simulink model "usrmpc"  (R2018b)
settings: Solver=VariableStepAuto  StartTime=0.0  StopTime=10.0  RelTol=1e-3
settings Model: Creator=dongdaming  LastModifiedBy=dongdaming

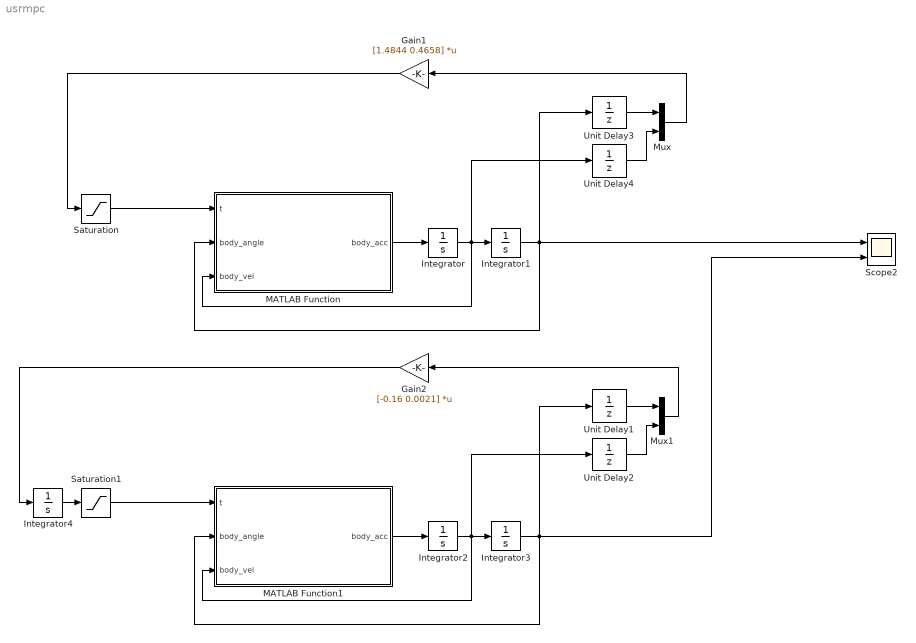
== system usrmpc ==
  Gain1 : Gain  Gain=[1.4844 0.4658]  Multiplication=Matrix(K*u)
  Gain2 : Gain  Gain=[-0.16 0.0021]  Multiplication=Matrix(K*u)
  Integrator : Integrator
  Integrator1 : Integrator  InitialCondition=pi/3  LimitOutput=on  UpperSaturationLimit=pi  LowerSaturationLimit=-pi
  Integrator2 : Integrator
  Integrator3 : Integrator  InitialCondition=pi/3  LimitOutput=on  UpperSaturationLimit=pi  LowerSaturationLimit=-pi
  Integrator4 : Integrator
  MATLAB Function : MATLAB Function  TreatAsAtomicUnit=on
  MATLAB Function1 : MATLAB Function  TreatAsAtomicUnit=on
  Mux : Mux  Inputs=2
  Mux1 : Mux  Inputs=2
  Saturation : Saturate  UpperLimit=1.4  LowerLimit=-1.4
  Saturation1 : Saturate  UpperLimit=1.4  LowerLimit=-1.4
  Scope2 : Scope  NumInputPorts=2
  Unit Delay{1..4} (4 alike) : UnitDelay  InitialCondition=pi/3  SampleTime=0.002
  wires:
  Saturation/1 -> MATLAB Function/1(t)
  Integrator1/1 -> MATLAB Function/2(body_angle), Scope2/1, Unit Delay3/1
  Integrator/1 -> Unit Delay4/1, MATLAB Function/3(body_vel), Integrator1/1
  MATLAB Function/1(body_acc) -> Integrator/1
  Mux/1 -> Gain1/1
  Unit Delay4/1 -> Mux/2
  Unit Delay3/1 -> Mux/1
  Gain1/1 -> Saturation/1
  Unit Delay1/1 -> Mux1/1
  Unit Delay2/1 -> Mux1/2
  MATLAB Function1/1(body_acc) -> Integrator2/1
  Integrator2/1 -> Integrator3/1, MATLAB Function1/3(body_vel), Unit Delay2/1
  Integrator3/1 -> Unit Delay1/1, Scope2/2, MATLAB Function1/2(body_angle)
  Saturation1/1 -> MATLAB Function1/1(t)
  Integrator4/1 -> Saturation1/1
  Gain2/1 -> Integrator4/1
  Mux1/1 -> Gain2/1

== matlab function usrmpc/MATLAB Function1 ==
  data: t input; body_acc output; body_angle input; body_vel input
function body_acc = fcn(t,body_angle,body_vel)
body_acc=(+1429.48*sin(body_angle)-1215.55*t-2083.85*t*cos(body_angle)-3.87597*sin(2*body_angle)*body_vel^2)/(2.91931+cos(body_angle)^2+8.75194*sin(body_angle)^2);

== matlab function usrmpc/MATLAB Function ==
  data: t input; body_acc output; body_angle input; body_vel input
function body_acc = fcn(t,body_angle,body_vel)
body_acc=(+1429.48*sin(body_angle)-1215.55*t-2083.85*t*cos(body_angle)-3.87597*sin(2*body_angle)*body_vel^2)/(2.91931+cos(body_angle)^2+8.75194*sin(body_angle)^2);
